simulink model "pitchratecommand"  (R2022a)
settings: Solver=VariableStepAuto  StartTime=0.0  StopTime=25  RelTol=1e-3
values from neighbouring files (symbols this model uses):
  A_red = [  -0.3190      0.9509 ... (first row only)    [chapter7.m]    (also in untitled3.m)
  B_red = [ -0.0007 ... (first row only)    [chapter7.m]    (also in untitled3.m)
  C_red = [57.2958, 0; 0, 57.2958]    [chapter7.m]    (also in untitled3.m)
  D_red = [0; 0]    [chapter7.m]    (also in untitled3.m)
  K_red = place(A_red, B_red, p)    [chapter7.m]
settings Model: Creator=mihai  LastModifiedBy=mihai

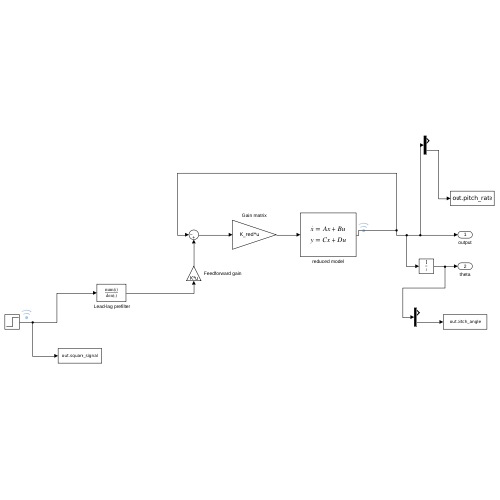
[thumbnail: Simulink's stored preview of the top-level diagram]
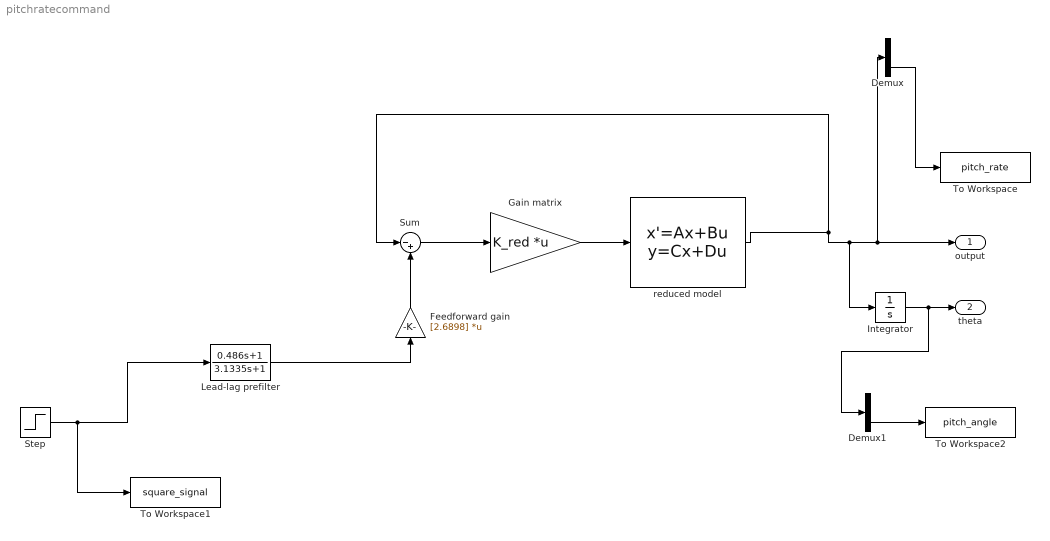
== system pitchratecommand ==
  " Lead-lag prefilter" : TransferFcn  Numerator=[0.486, 1]  Denominator=[3.1335, 1]
  Demux : Demux  Outputs=2
  Demux1 : Demux  Outputs=2
  Feedforward gain : Gain  Gain=[2.6898]  Multiplication=Matrix(K*u)
  Gain matrix : Gain  Gain=K_red  Multiplication=Matrix(K*u)
  Integrator : Integrator
  Step : Step  OutDataTypeStr=Inherit: Inherit via back propagation  SampleTime=0
  Sum : Sum  Inputs=|-+
  To Workspace : ToWorkspace  VariableName=pitch_rate  SaveFormat=Timeseries  SampleTime=-1
  To Workspace1 : ToWorkspace  VariableName=square_signal  SaveFormat=Timeseries  SampleTime=-1
  To Workspace2 : ToWorkspace  VariableName=pitch_angle  SaveFormat=Timeseries  SampleTime=-1
  reduced model : StateSpace  A=A_red  B=B_red  C=C_red  D=D_red  InitialCondition=0
  output : Outport
  theta : Outport  Port=2
  wires:
  Gain matrix/1 -> reduced model/1
  Sum/1 -> Gain matrix/1
  Step/1 -> To Workspace1/1, " Lead-lag prefilter"/1
  " Lead-lag prefilter"/1 -> Feedforward gain/1
  Feedforward gain/1 -> Sum/2
  Integrator/1 -> Demux1/1, theta/1
  reduced model/1 -> Integrator/1, Demux/1, output/1, Sum/1
  Demux/2 -> To Workspace/1
  Demux1/2 -> To Workspace2/1
